simulink model "sis"  (R2012b)
settings: Solver=ode45  StartTime=0.0  StopTime=2.5  RelTol=1e-3
settings Model: Creator=Alunos  LastModifiedBy=Alunos

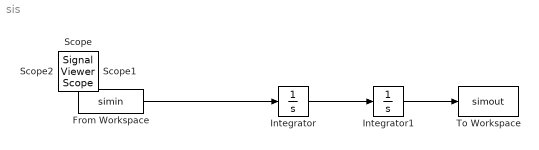
== system sis ==
  From Workspace : FromWorkspace  VariableName=simin  SampleTime=0  OutputAfterFinalValue=Setting to zero
  Integrator : Integrator
  Integrator1 : Integrator
  To Workspace : ToWorkspace  VariableName=simout  SampleTime=-1  SaveFormat=Timeseries
  Scope : SignalViewerScope  IOType=viewer  RefreshTime=0.035000
  Scope1 : SignalViewerScope  IOType=viewer  RefreshTime=0.035000
  Scope2 : SignalViewerScope  IOType=viewer  RefreshTime=0.035000
      settings: SaveName=ScopeData2
  wires:
  Integrator/1 -> Integrator1/1
  From Workspace/1 -> Integrator/1
  Integrator1/1 -> To Workspace/1
